simulink model "triHmotneBody"  (R2020b)
settings: Solver=FixedStepAuto  StartTime=0.0  StopTime=10.0  FixedStep=stepSize  RelTol=1e-3
values from neighbouring files (symbols this model uses):
  b = 0    [triHmotneBodyM.m]
  F = 0    [triHmotneBodyM.m]
  k = 1    [triHmotneBodyM.m]
  m = 1    [triHmotneBodyM.m]
  x1_0 = 0    [triHmotneBodyM.m]
  x1d_0 = 0    [triHmotneBodyM.m]
  x2_0 = 1    [triHmotneBodyM.m]
  x2d_0 = 0    [triHmotneBodyM.m]
  x3_0 = 2    [triHmotneBodyM.m]
  x3d_0 = 0    [triHmotneBodyM.m]
settings Model: Creator=ADMIN  LastModifiedBy=Admin

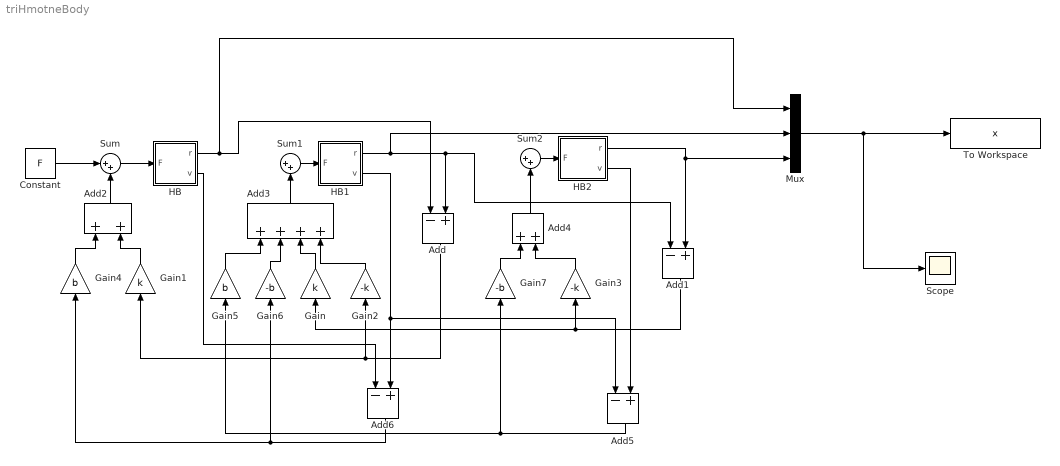
== system triHmotneBody ==
  Add{,1,5..6} (4 alike) : Sum  Inputs=-+
  Add2 : Sum
  Add3 : Sum  Inputs=++++
  Add4 : Sum
  Constant : Constant  Value=F
  Gain : Gain  Gain=k
  Gain1 : Gain  Gain=k
  Gain2 : Gain  Gain=-k
  Gain3 : Gain  Gain=-k
  Gain4 : Gain  Gain=b
  Gain5 : Gain  Gain=b
  Gain6 : Gain  Gain=-b
  Gain7 : Gain  Gain=-b
  HB : Subsystem
  HB1 : Subsystem
  HB2 : Subsystem
  Mux : Mux  Inputs=3
  Scope : Scope
  Sum : Sum  Inputs=|++
  Sum1 : Sum  Inputs=|++
  Sum2 : Sum  Inputs=|++
  To Workspace : ToWorkspace  VariableName=x  SaveFormat=Structure With Time  SampleTime=-1
  wires:
  Sum1/1 -> HB1/1(F)
  Sum2/1 -> HB2/1(F)
  Sum/1 -> HB/1(F)
  Constant/1 -> Sum/1
  HB/1(r) -> Add/1, Mux/1
  HB2/1(r) -> Mux/3, Add1/2
  HB1/1(r) -> Add1/1, Add/2, Mux/2
  Add1/1 -> Gain/1, Gain3/1
  Add/1 -> Gain1/1, Gain2/1
  Add2/1 -> Sum/2
  Gain1/1 -> Add2/2
  Gain4/1 -> Add2/1
  Add3/1 -> Sum1/2
  Gain2/1 -> Add3/4
  Gain/1 -> Add3/3
  Gain5/1 -> Add3/1
  Gain6/1 -> Add3/2
  Add4/1 -> Sum2/2
  Gain7/1 -> Add4/1
  Gain3/1 -> Add4/2
  HB2/2(v) -> Add5/2
  HB1/2(v) -> Add6/2, Add5/1
  HB/2(v) -> Add6/1
  Add6/1 -> Gain6/1, Gain4/1
  Add5/1 -> Gain5/1, Gain7/1
  Mux/1 -> To Workspace/1, Scope/1

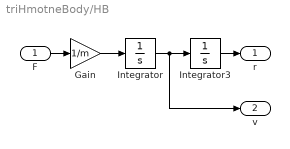
== system triHmotneBody/HB ==
  F : Inport
  Gain : Gain  Gain=1/m
  Integrator : Integrator  InitialCondition=x1d_0
  Integrator3 : Integrator  InitialCondition=x1_0
  r : Outport
  v : Outport  Port=2
  wires:
  Gain/1 -> Integrator/1
  F/1 -> Gain/1
  Integrator/1 -> v/1, Integrator3/1
  Integrator3/1 -> r/1

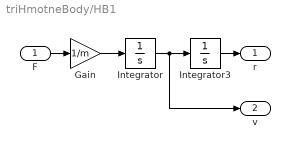
== system triHmotneBody/HB1 ==
  F : Inport
  Gain : Gain  Gain=1/m
  Integrator : Integrator  InitialCondition=x2d_0
  Integrator3 : Integrator  InitialCondition=x2_0
  r : Outport
  v : Outport  Port=2
  wires:
  Gain/1 -> Integrator/1
  F/1 -> Gain/1
  Integrator/1 -> v/1, Integrator3/1
  Integrator3/1 -> r/1

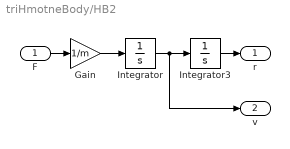
== system triHmotneBody/HB2 ==
  F : Inport
  Gain : Gain  Gain=1/m
  Integrator : Integrator  InitialCondition=x3d_0
  Integrator3 : Integrator  InitialCondition=x3_0
  r : Outport
  v : Outport  Port=2
  wires:
  Gain/1 -> Integrator/1
  F/1 -> Gain/1
  Integrator/1 -> v/1, Integrator3/1
  Integrator3/1 -> r/1
